simulink model "ASKzhangqingzhuo6_5"  (Simulink 5.0)
settings: Solver=ode45  StartTime=0.0  StopTime=10.0  RelTol=1e-3
libraries: dsparch4 x3, commsink2 x2, commchan2 x1, commrandsrc2 x1
settings Model: LastModifiedBy=lenovo

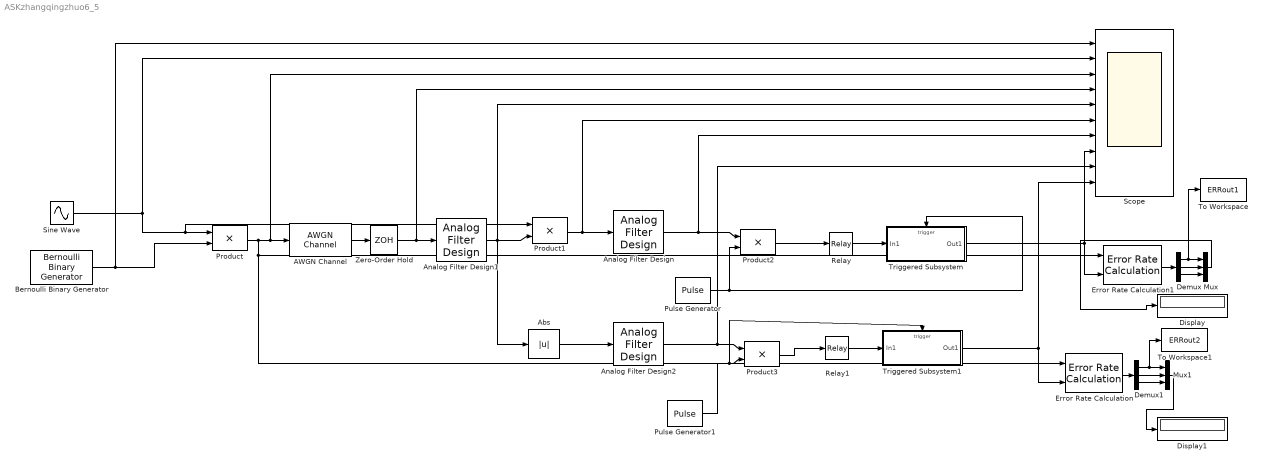
== system ASKzhangqingzhuo6_5 ==
  AWGN Channel : commchan2/AWGN Channel  seed=67  noiseMode="Signal to noise ratio  (SNR)"  EsNodB=10  SNRdB=10  Ps=1  Tsym=1  variance=1
  Abs : Abs  SaturateOnIntegerOverflow=on
  Analog Filter Design : dsparch4/Analog Filter Design  method=Butterworth  filttype=Lowpass  N=8  Wlo=2*pi*5  Whi=80  Rp=2  Rs=40
  Analog Filter Design1 : dsparch4/Analog Filter Design  method=Butterworth  filttype=Bandpass  N=8  Wlo=2*pi*18  Whi=2*pi*22  Rp=2  Rs=40
  Analog Filter Design2 : dsparch4/Analog Filter Design  method=Butterworth  filttype=Lowpass  N=8  Wlo=2*pi*5  Whi=80  Rp=2  Rs=40
  Bernoulli Binary Generator : commrandsrc2/Bernoulli Binary Generator  P=0.5  seed=61  Ts=0.5  frameBased=off  sampPerFrame=1  orient=off
  Demux : Demux  Outputs=3
  Demux1 : Demux  Outputs=3
  Display : Display
  Display1 : Display
  Error Rate Calculation : commsink2/Error Rate Calculation  N=0  st_delay=0  cp_mode=Entire frame  subframe=[]  PMode=Port  WsName=ErrorVec  RsMode2=off  stop=off  numErr=100  maxBits=1e6
  Error Rate Calculation1 : commsink2/Error Rate Calculation  N=0  st_delay=0  cp_mode=Entire frame  subframe=[]  PMode=Port  WsName=ErrorVec  RsMode2=off  stop=off  numErr=100  maxBits=1e6
  Mux : Mux  Inputs=3
  Mux1 : Mux  Inputs=3
  Product{,1..3} (4 alike) : Product  SaturateOnIntegerOverflow=on
  Pulse Generator : DiscretePulseGenerator  Period=10  PulseWidth=5  SampleTime=1/500
  Pulse Generator1 : DiscretePulseGenerator  Period=10  PulseWidth=5  SampleTime=1/500
  Relay : Relay  OnSwitchValue=0.2  OffSwitchValue=0.2  ShowAdditionalParam=on
  Relay1 : Relay  OnSwitchValue=0.3  OffSwitchValue=0.3  ShowAdditionalParam=on
  Scope : Scope  NumInputPorts=10
      settings: YMin=-2~-2~-2~-2~-2~-2~-2~-2~-2~-2  YMax=2~2~2~2~2~2~2~2~2~2
  Sine Wave : Sin  Frequency=2*pi*20  SampleTime=1/500
  To Workspace : ToWorkspace  VariableName=ERRout1  SampleTime=-1  SaveFormat=Structure
  To Workspace1 : ToWorkspace  VariableName=ERRout2  SampleTime=-1  SaveFormat=Structure
  Triggered Subsystem : Subsystem  TreatAsAtomicUnit=on
  Triggered Subsystem1 : Subsystem  TreatAsAtomicUnit=on
  Zero-Order Hold : ZeroOrderHold  SampleTime=0.01
  wires:
  Bernoulli Binary Generator/1 -> Scope/1, Product/2
  Abs/1 -> Analog Filter Design2/1
  Product2/1 -> Relay/1
  Relay/1 -> Triggered Subsystem/1(In1)
  Relay1/1 -> Triggered Subsystem1/1(In1)
  Pulse Generator/1 -> Triggered Subsystem/Trigger, Product2/2
  Triggered Subsystem/1(Out1) -> Scope/8, Error Rate Calculation1/2
  Product3/1 -> Relay1/1
  Triggered Subsystem1/1(Out1) -> Scope/10, Error Rate Calculation/2
  Pulse Generator1/1 -> Triggered Subsystem1/Trigger, Product3/2
  Error Rate Calculation1/1 -> Demux/1
  Demux/2 -> Mux/2
  Demux/3 -> Mux/3
  Demux1/1 -> Mux1/1, To Workspace1/1
  Demux1/2 -> Mux1/2
  Demux1/3 -> Mux1/3
  Error Rate Calculation/1 -> Demux1/1
  Demux/1 -> Mux/1, To Workspace/1
  Mux1/1 -> Display1/1
  Mux/1 -> Display/1
  AWGN Channel/1 -> Zero-Order Hold/1
  Analog Filter Design2/1 -> Scope/9, Product3/1
  Analog Filter Design/1 -> Scope/7, Product2/1
  Product1/1 -> Analog Filter Design/1, Scope/6
  Analog Filter Design1/1 -> Abs/1, Scope/5, Product1/2
  Zero-Order Hold/1 -> Analog Filter Design1/1, Scope/4
  Product/1 -> AWGN Channel/1, Scope/3, Error Rate Calculation1/1, Error Rate Calculation/1
  Sine Wave/1 -> Product/1, Product1/1, Scope/2

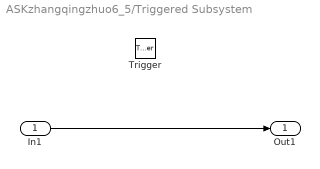
== system ASKzhangqingzhuo6_5/Triggered Subsystem ==
  In1 : Inport
  Trigger : TriggerPort
  Out1 : Outport
  wires:
  In1/1 -> Out1/1

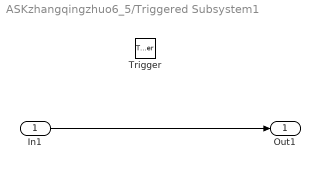
== system ASKzhangqingzhuo6_5/Triggered Subsystem1 ==
  In1 : Inport
  Trigger : TriggerPort
  Out1 : Outport
  wires:
  In1/1 -> Out1/1
